simulink model "program2"  (Simulink 9.0)
settings: Solver=VariableStepAuto  StartTime=0.0  StopTime=10.0  RelTol=1e-3
values from neighbouring files (symbols this model uses):
  L = [1 -2 4]    [ModelDD.m]
libraries: roblocks x2, simulink x1
settings Model: Creator=ACER  LastModifiedBy=ACER
settings DataIOCC: SaveFormat=Dataset  ReturnWorkspaceOutputs=on
settings OptimizationCC: LifeSpan=auto
settings DebuggingCC: UnderspecifiedInitializationDetection=Simplified  MergeDetectMultiDrivingBlocksExec=error  SFUnexpectedBacktrackingDiag=error  SFNoUnconditionalDefaultTransitionDiag=error  SFExecutionAtInitializationDiag=warning
settings HardwareCC: ProdBitPerPointer=64  ProdBitPerSizeT=64  ProdBitPerPtrDiffT=64  ProdLargestAtomicFloat=Float  ProdIntDivRoundTo=Zero  ProdEndianess=LittleEndian  ProdWordSize=64  ProdHWDeviceType=Intel->x86-64 (Windows64)
settings ModelReferenceCC: PropagateSignalLabelsOutOfModel=on
settings SFSimCC: SimUseLocalCustomCode=on
settings RTWCC: RTWUseLocalCustomCode=on
settings CodeAppCC: StateflowObjectComments=off
settings GRTTargetCC: TargetLangStandard=C99 (ISO)
settings ConfigComp: CovMetricSettings=dwe  CovHtmlReporting=off  CovSaveCumulativeToWorkspaceVar=off  CovSaveSingleToWorkspaceVar=off  CovExternalEMLEnable=on

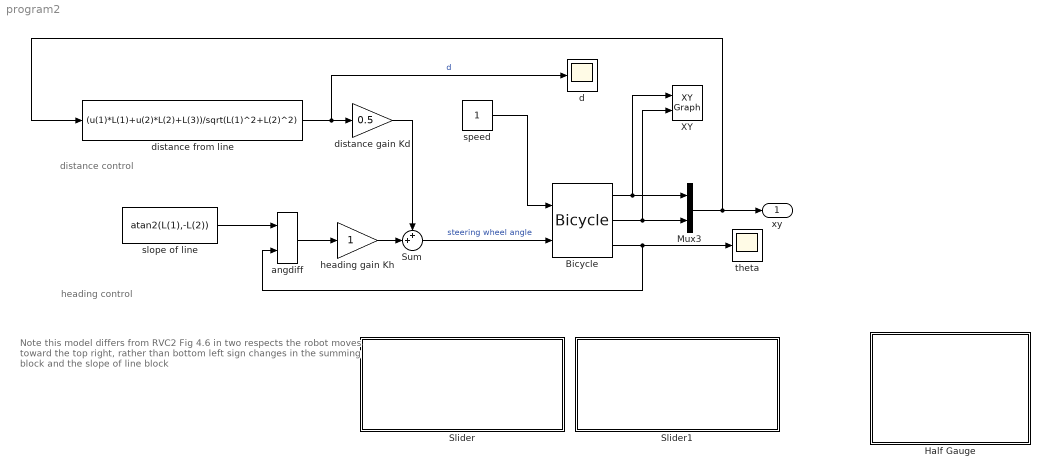
== system program2 ==
  note: Note this model differs from RVC2 Fig 4.6 in two respects
      | the robot moves toward the top right, rather than bottom left
      | sign changes in the summing block and the slope of line block
  note: heading control
  note: distance control
  Bicycle : roblocks/Vehicles/Bicycle  vlim=1  accel=1  alim=1  steer_rate=Inf  L=1  x0=x0
  Half Gauge : Subsystem  DialogController=hmiCreateDDGDialog  DialogControllerArgs=DataTag0  IsWebBlock=on  mask(MWDashboardBlock){webBlockId=21cc0dd8-7c39-4ee2-9863-f6653e26bb66, webBlockType=semicirculargauge, ShowInLibBrowser=on, ShowInitialText=on, HMISrcModelName=program2}
      mask prompts: webBlockId "WebBlock Id"; webBlockType "WebBlock Type"; HMISrcModelName "Source Model"
      mask help: Display an input value on a semicircular scale.
      mask Help: helpview([docroot '/mapfiles/simulink.map'], 'hmi_half_gauge')
      mask Display:
      | if strcmp(get_param(bdroot(gcb),'BlockDiagramType'),'library')
      |  image([(matlabroot) '/toolbox/simulink/hmi/icons/SemiCircularGauge.png'])
      | end
  Mux3 : Mux  Inputs=2
  Slider : Subsystem  DialogController=hmiCreateDDGDialog  DialogControllerArgs=DataTag1  IsWebBlock=on  mask(MWDashboardBlock){webBlockId=aa4f79a0-7ec3-4d50-a6f7-a1dd725aba8a, webBlockType=slider, ShowInLibBrowser=on, ShowInitialText=on, HMISrcModelName=program2}
      mask prompts: webBlockId "WebBlock Id"; webBlockType "WebBlock Type"; HMISrcModelName "Source Model"
      mask help: Set value to tune parameters or variables.
      mask Help: helpview([docroot '/mapfiles/simulink.map'], 'hmi_slider')
      mask Display:
      | if strcmp(get_param(bdroot(gcb),'BlockDiagramType'),'library')
      |  image([(matlabroot) '/toolbox/simulink/hmi/icons/Slider.png'])
      | end
  Slider1 : Subsystem  DialogController=hmiCreateDDGDialog  DialogControllerArgs=DataTag2  IsWebBlock=on  mask(MWDashboardBlock){webBlockId=f6e67e94-80f7-4839-a95b-4aaf55e44598, webBlockType=slider, ShowInLibBrowser=on, ShowInitialText=on, HMISrcModelName=program2}
      mask prompts: webBlockId "WebBlock Id"; webBlockType "WebBlock Type"; HMISrcModelName "Source Model"
      mask help: Set value to tune parameters or variables.
      mask Help: helpview([docroot '/mapfiles/simulink.map'], 'hmi_slider')
      mask Display:
      | if strcmp(get_param(bdroot(gcb),'BlockDiagramType'),'library')
      |  image([(matlabroot) '/toolbox/simulink/hmi/icons/Slider.png'])
      | end
  Sum : Sum  Inputs=++|
  XY : simulink/Sinks/XY Graph  xmin=-10  xmax=10  ymin=-10  ymax=10  st=-1
  angdiff : roblocks/Toolbox/angdiff
  d : Scope
  distance from line : Fcn  Expr=(u(1)*L(1)+u(2)*L(2)+L(3))/sqrt(L(1)^2+L(2)^2)
  distance gain Kd : Gain  Gain=0.5
  heading gain Kh : Gain
  slope of line : Constant  Value=atan2(L(1),-L(2))
  speed : Constant  VectorParams1D=off  SampleTime=0.02
  theta : Scope
  xy : Outport  VectorParamsAs1DForOutWhenUnconnected=off
  wires:
  slope of line/1 -> angdiff/1
  Bicycle/1 -> XY/1, Mux3/1
  Sum/1 -> Bicycle/2  "steering wheel angle"
  heading gain Kh/1 -> Sum/2
  Bicycle/2 -> XY/2, Mux3/2
  distance from line/1 -> distance gain Kd/1, d/1  "d"
  speed/1 -> Bicycle/1
  distance gain Kd/1 -> Sum/1
  Bicycle/3 -> angdiff/2, theta/1
  Mux3/1 -> distance from line/1, xy/1
  angdiff/1 -> heading gain Kh/1

== system program2/Half Gauge ==

== system program2/Slider ==

== system program2/Slider1 ==
